simulink model "example_Resident_Data"  (R2018b)
settings: Solver=ode45  StartTime=0.0  StopTime=1*24*3600  MaxStep=600  RelTol=1e-4  AbsTol=1e-6  EnableMultiTasking=on
libraries: simulink x3, carnot x1
settings Model: Creator=drhf  LastModifiedBy=drhf
settings SolverCC: AutoScaleAbsTol=off  ZeroCrossAlgorithm=Adaptive
settings DataIOCC: LimitDataPoints=on  SaveFormat=Array
settings OptimizationCC: ExpressionDepthLimit=2147483647  LifeSpan=inf
settings DebuggingCC: UnderspecifiedInitializationDetection=Classic  MergeDetectMultiDrivingBlocksExec=none  SolverPrmCheckMsg=warning  StateNameClashWarn=warning  SFUnexpectedBacktrackingDiag=warning  SFNoUnconditionalDefaultTransitionDiag=warning  SFExecutionAtInitializationDiag=none
settings HardwareCC: ProdBitPerPointer=32  ProdBitPerSizeT=32  ProdBitPerPtrDiffT=32  ProdLargestAtomicFloat=None  ProdIntDivRoundTo=Undefined  ProdEndianess=Unspecified  ProdWordSize=32  ProdHWDeviceType=32-bit Generic
settings ModelReferenceCC: PropagateSignalLabelsOutOfModel=off
settings SFSimCC: SimUseLocalCustomCode=off
settings RTWCC: RTWUseLocalCustomCode=off
settings CodeAppCC: StateflowObjectComments=on
settings GRTTargetCC: TargetLangStandard=C89/C90 (ANSI)  GeneratePreprocessorConditionals=Disable all  CombineOutputUpdateFcns=off  GRTInterface=on
settings ConfigComp: CovMetricSettings=dw  CovHtmlReporting=on  CovSaveCumulativeToWorkspaceVar=on  CovSaveSingleToWorkspaceVar=on  CovExternalEMLEnable=off

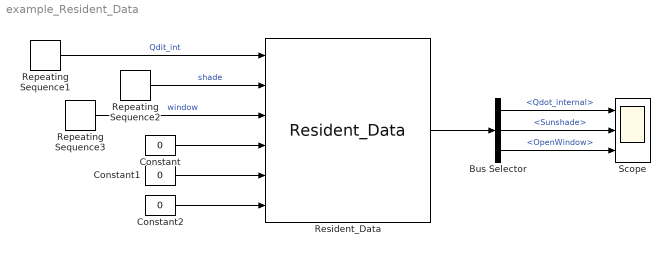
== system example_Resident_Data ==
  Bus Selector : BusSelector  OutputSignals=Qdot_internal,Sunshade,OpenWindow
  Constant : Constant  Value=0
  Constant1 : Constant  Value=0
  Constant2 : Constant  Value=0
  Repeating Sequence1 : simulink/Sources/Repeating Sequence  rep_seq_t="[0  12 24]*3600"  rep_seq_y=[100 500 100]
  Repeating Sequence2 : simulink/Sources/Repeating Sequence  rep_seq_t="[0  12 24]*3600"  rep_seq_y=[0 1 0]
  Repeating Sequence3 : simulink/Sources/Repeating Sequence  rep_seq_t=[0 8 9 10 12 18 19 20 24]*3600  rep_seq_y=[0 0 1 1 0 0 1 1 0]
  Resident_Data : carnot/Load/Houses/Resident_Data  CalcAirComp=on
      settings: SourceProductName=Carnot
  Scope : Scope  NumInputPorts=3
  wires:
  Resident_Data/1 -> Bus Selector/1
  Bus Selector/2 -> Scope/2  "<Sunshade>"
  Bus Selector/1 -> Scope/1  "<Qdot_internal>"
  Bus Selector/3 -> Scope/3  "<OpenWindow>"
  Repeating Sequence1/1 -> Resident_Data/1  "Qdit_int"
  Repeating Sequence2/1 -> Resident_Data/2  "shade"
  Repeating Sequence3/1 -> Resident_Data/3  "window"
  Constant/1 -> Resident_Data/4
  Constant1/1 -> Resident_Data/5
  Constant2/1 -> Resident_Data/6
